simulink model "digital_control"  (R2017b)
settings: Solver=VariableStepAuto  StartTime=0.0  StopTime=15  RelTol=1e-3
values from neighbouring files (symbols this model uses):
  T = diff(T)    [process.m]    (also in script.m = data.Time_s_)
undefined symbols (not defined in the file or in its folder): dC, dP, P, sA, sB, sC, sD
libraries: dspsigops x4
settings Model: Creator=e25756  LastModifiedBy=qlong1505

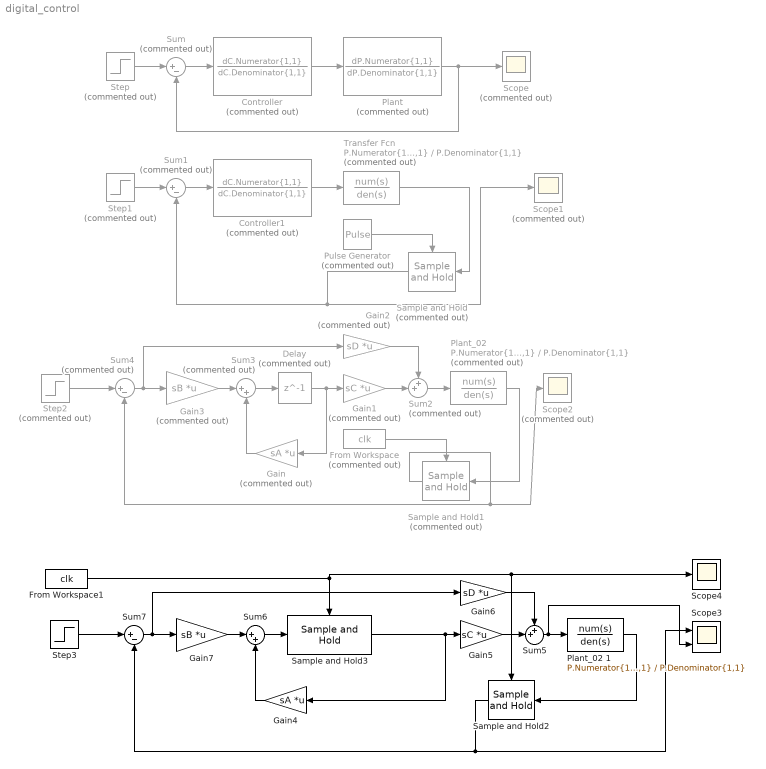
== system digital_control ==
  Controller : DiscreteTransferFcn  Commented=on  Numerator=dC.Numerator{1,1}  Denominator=dC.Denominator{1,1}  SampleTime=T
  Controller1 : DiscreteTransferFcn  Commented=on  Numerator=dC.Numerator{1,1}  Denominator=dC.Denominator{1,1}  SampleTime=T
  Delay : Delay  Commented=on  DelayLength=1  SampleTime=T
  From Workspace : FromWorkspace  Commented=on  VariableName=clk  SampleTime=T/2  Interpolate=off  OutputAfterFinalValue=Holding final value
  From Workspace1 : FromWorkspace  VariableName=clk  SampleTime=T/128  Interpolate=off  OutputAfterFinalValue=Holding final value
  Gain : Gain  Commented=on  Gain=sA  Multiplication=Matrix(K*u)
  Gain1 : Gain  Commented=on  Gain=sC  Multiplication=Matrix(K*u)
  Gain2 : Gain  Commented=on  Gain=sD  Multiplication=Matrix(K*u)
  Gain3 : Gain  Commented=on  Gain=sB  Multiplication=Matrix(K*u)
  Gain4 : Gain  Gain=sA  Multiplication=Matrix(K*u)
  Gain5 : Gain  Gain=sC  Multiplication=Matrix(K*u)
  Gain6 : Gain  Gain=sD  Multiplication=Matrix(K*u)
  Gain7 : Gain  Gain=sB  Multiplication=Matrix(K*u)
  Plant : DiscreteTransferFcn  Commented=on  Numerator=dP.Numerator{1,1}  Denominator=dP.Denominator{1,1}  SampleTime=T
  "Plant_02 " : TransferFcn  Commented=on  Numerator=P.Numerator{1,1}  Denominator=P.Denominator{1,1}
  Plant_02 1 : TransferFcn  Numerator=P.Numerator{1,1}  Denominator=P.Denominator{1,1}
  Pulse Generator : DiscretePulseGenerator  Commented=on  PulseType=Time based  Period=T  PulseWidth=50
  Sample and Hold : dspsigops/Sample and Hold  Commented=on  trig=Rising edge  initCond=0  latchinput=off
  Sample and Hold1 : dspsigops/Sample and Hold  Commented=on  trig=Rising edge  initCond=0  latchinput=off
  Sample and Hold2 : dspsigops/Sample and Hold  trig=Rising edge  initCond=0  latchinput=off
  Sample and Hold3 : dspsigops/Sample and Hold  trig=Rising edge  initCond=0  latchinput=on
  Scope : Scope  Commented=on
  Scope1 : Scope  Commented=on
  Scope2 : Scope  Commented=on
  Scope3 : Scope  NumInputPorts=2
  Scope4 : Scope
  Step : Step  Commented=on  Time=0  SampleTime=0
  Step1 : Step  Commented=on  Time=0  SampleTime=0
  Step2 : Step  Commented=on  Time=0  SampleTime=0
  Step3 : Step  Time=0  SampleTime=0
  Sum : Sum  Commented=on  Inputs=|+-
  Sum1 : Sum  Commented=on  Inputs=|+-
  Sum2 : Sum  Commented=on  Inputs=++|
  Sum3 : Sum  Commented=on  Inputs=|++
  Sum4 : Sum  Commented=on  Inputs=|+-
  Sum5 : Sum  Inputs=++|
  Sum6 : Sum  Inputs=|++
  Sum7 : Sum  Inputs=|+-
  Transfer Fcn : TransferFcn  Commented=on  Numerator=P.Numerator{1,1}  Denominator=P.Denominator{1,1}
  wires:
  Sum/1 -> Controller/1
  Step/1 -> Sum/1
  Controller/1 -> Plant/1
  Plant/1 -> Scope/1, Sum/2
  Transfer Fcn/1 -> Sample and Hold/1
  Controller1/1 -> Transfer Fcn/1
  Step1/1 -> Sum1/1
  Sum1/1 -> Controller1/1
  Sample and Hold/1 -> Sum1/2, Scope1/1
  Pulse Generator/1 -> Sample and Hold/Trigger
  Gain2/1 -> Sum2/1
  Delay/1 -> Gain1/1, Gain/1
  Gain3/1 -> Sum3/1
  Gain/1 -> Sum3/2
  Sum3/1 -> Delay/1
  Gain1/1 -> Sum2/2
  Sum4/1 -> Gain3/1, Gain2/1
  Sum2/1 -> "Plant_02 "/1
  Sample and Hold1/1 -> Scope2/1, Sum4/2
  "Plant_02 "/1 -> Sample and Hold1/1
  Step2/1 -> Sum4/1
  From Workspace/1 -> Sample and Hold1/Trigger
  Step3/1 -> Sum7/1
  Plant_02 1/1 -> Sample and Hold2/1
  Gain4/1 -> Sum6/2
  From Workspace1/1 -> Scope4/1, Sample and Hold2/Trigger, Sample and Hold3/Trigger
  Sum7/1 -> Gain7/1, Gain6/1
  Sum6/1 -> Sample and Hold3/1
  Gain5/1 -> Sum5/2
  Sum5/1 -> Scope3/2, Plant_02 1/1
  Gain7/1 -> Sum6/1
  Gain6/1 -> Sum5/1
  Sample and Hold2/1 -> Scope3/1, Sum7/2
  Sample and Hold3/1 -> Gain5/1, Gain4/1
